simulink model "teste2clana"  (R2014a)
settings: Solver=ode3  StartTime=0.0  StopTime=40  FixedStep=0.001  RelTol=1e-3
settings Model: Creator=andre  LastModifiedBy=andre

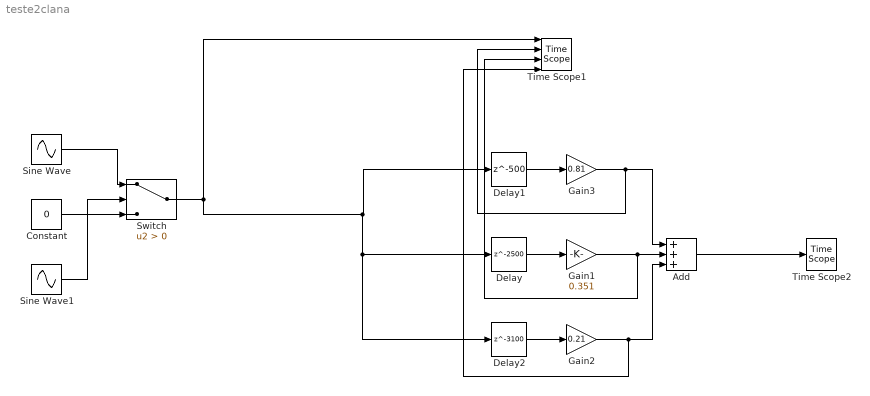
== system teste2clana ==
  Add : Sum  Inputs=+++
  Constant : Constant  Value=0
  Delay : Delay  DelayLength=2500
  Delay1 : Delay  DelayLength=500
  Delay2 : Delay  DelayLength=3100
  Gain1 : Gain  Gain=0.351
  Gain2 : Gain  Gain=0.21
  Gain3 : Gain  Gain=0.81
  Sine Wave : Sin  Frequency=5  SampleTime=0
  Sine Wave1 : Sin  SampleTime=0
  Switch : Switch  Criteria=u2 > Threshold
  Time Scope1 : TimeScope  NumInputPorts=4  DefaultConfigurationName=spbscopes.TimeScopeBlockCfg
  Time Scope2 : TimeScope  DefaultConfigurationName=spbscopes.TimeScopeBlockCfg
  wires:
  Gain1/1 -> Time Scope1/3, Add/2
  Gain3/1 -> Time Scope1/2, Add/1
  Sine Wave/1 -> Switch/1
  Sine Wave1/1 -> Switch/2
  Constant/1 -> Switch/3
  Gain2/1 -> Time Scope1/4, Add/3
  Delay2/1 -> Gain2/1
  Delay1/1 -> Gain3/1
  Delay/1 -> Gain1/1
  Add/1 -> Time Scope2/1
  Switch/1 -> Delay2/1, Delay/1, Delay1/1, Time Scope1/1
